simulink model "DCV_tester"  (R2024b)
settings: Solver=FixedStepAuto  StartTime=0.0  StopTime=2  FixedStep=0.01  RelTol=1e-3
settings Model: Creator=Emil  LastModifiedBy=Emil

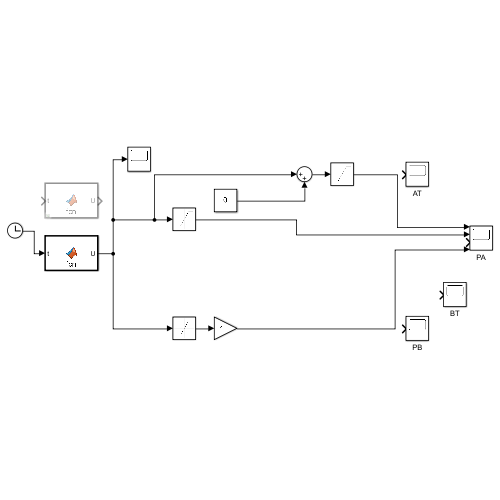
[thumbnail: Simulink's stored preview of the top-level diagram]
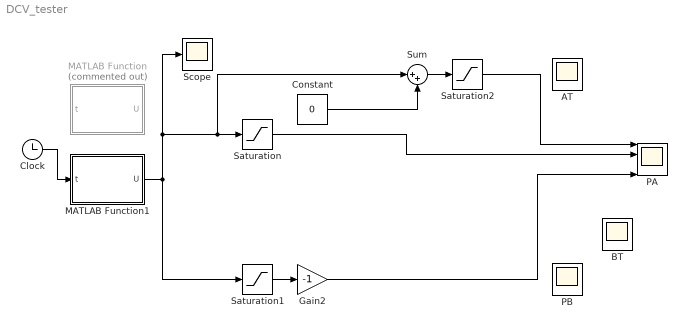
== system DCV_tester ==
  AT : Scope
  BT : Scope
  Clock : Clock
  Constant : Constant  Value=0
  Gain2 : Gain  Gain=-1
  MATLAB Function : MATLAB Function  Commented=on  TreatAsAtomicUnit=on
  MATLAB Function1 : MATLAB Function  TreatAsAtomicUnit=on
  PA : Scope  NumInputPorts=4
  PB : Scope
  Saturation : Saturate  UpperLimit=1  LowerLimit=0
  Saturation1 : Saturate  UpperLimit=0  LowerLimit=-1
  Saturation2 : Saturate  UpperLimit=1  LowerLimit=0
  Scope : Scope
  Sum : Sum  Inputs=|++
  wires:
  Clock/1 -> MATLAB Function1/1(t)
  MATLAB Function1/1(U) -> Saturation1/1, Scope/1, Sum/1, Saturation/1
  Saturation1/1 -> Gain2/1
  Saturation/1 -> PA/2
  Gain2/1 -> PA/4
  Sum/1 -> Saturation2/1
  Constant/1 -> Sum/2
  Saturation2/1 -> PA/1

== matlab function DCV_tester/MATLAB Function ==
  data: t input; U output
function U = fcn(t)
t_ramp = 1;
t_hold = 0.5;

if t < t_hold
    U = 0;
elseif t < t_ramp+t_hold
    U=1*(t-t_hold)/t_ramp;
elseif t < t_ramp+t_hold*2
    U=1;
elseif t < t_ramp*2+t_hold*2
    U=1-1*(t-t_ramp-t_hold*2)/t_ramp;
elseif t < t_ramp*2+t_hold*3
    U=0;
elseif t < t_ramp*3+t_hold*3
    U=-1*(t-t_ramp*2-t_hold*3)/t_ramp;
elseif t < t_ramp*3+t_hold*4
    U = -1;
elseif t < t_ramp*4+t_hold*4
    U=-1+1*(t-t_ramp*3-t_hold*4)/t_ramp;
else
    U = 0;
end

== matlab function DCV_tester/MATLAB Function1 ==
  data: t input; U output
function U = fcn(t)
t_ramp = 0.85;
t_hold = 0.15;

if t < t_ramp
   U = -1 + 1*t/t_ramp;
elseif t < t_ramp+t_hold*2
    U  = 0;
elseif t < t_ramp*2+t_hold*2
    U = 1*(t-t_ramp-t_hold*2)/t_ramp;
else 
    U = 0;
end
